simulink model "SEMD_E23_01_MDL"  (Simulink 7.9)
settings: Solver=ode45  StartTime=0.0  StopTime=tstop  MaxStep=0.1  RelTol=1e-3
values from neighbouring files (symbols this model uses):
  D = 0.9*D0    (= 0.03501)    [SEMD_E23_01.m]
  deriv = @(x,D) [      Xdot(x(1),x(2),x(3),D) ... (first row only)    [SEMD_E23_01.m]
  x0 = trim(mdl)    [SEMD_E23_01.m]
settings Model: Creator=jeff  LastModifiedBy=jeff

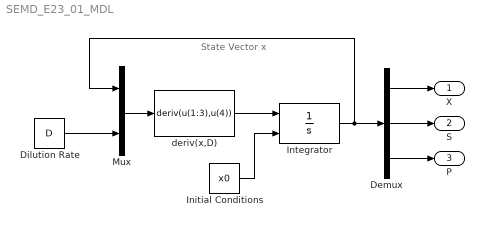
== system SEMD_E23_01_MDL ==
  note: State Vector x
  Demux : Demux  Outputs=3
  "Dilution Rate " : Constant  Value=D
  Initial Conditions : Constant  Value=x0  VectorParams1D=off
  Integrator : Integrator  InitialConditionSource=external  InitialCondition=x0  ContinuousStateAttributes={'X','S','P'}
  Mux : Mux  Inputs=2
  deriv(x,D) : MATLABFcn  MATLABFcn=deriv(u(1:3),u(4))
  X : Outport
  S : Outport  Port=2
  P : Outport  Port=3
  wires:
  "Dilution Rate "/1 -> Mux/2
  Initial Conditions/1 -> Integrator/2
  Mux/1 -> deriv(x,D)/1
  Integrator/1 -> Mux/1, Demux/1
  deriv(x,D)/1 -> Integrator/1
  Demux/1 -> X/1
  Demux/2 -> S/1
  Demux/3 -> P/1
